simulink model "controllReal"  (R2018a)
settings: Solver=VariableStepAuto  StartTime=0.0  StopTime=1000  RelTol=1e-3
values from neighbouring files (symbols this model uses):
  a = 0.17    [Lab1.m]
  A = 33    [Lab1.m]
  g = 981    [Lab1.m]
  h = 5:1:15    [Lab1.m]
  h0 = 3.2    [Lab1.m]
  hV = [1.826, 2.539, 3.452, 4.18, 4.99, 5.762, 6.665, 7.36, 8.193, 8.93, 9.66]    [Lab1.m]
  v = 1:1:10    [Lab1.m]
  vt = [21.18, 26.66 30.97, 34.28, 37.92, 39.73, 42.53, 45.45, 46.49, 47.67]    [Lab1.m]
undefined symbols (not defined in the file or in its folder): National_Instruments, PCI, sigbuilder_block
libraries: sldrtlib x2
settings Model: Creator=scofre-5  LastModifiedBy=scofre-5

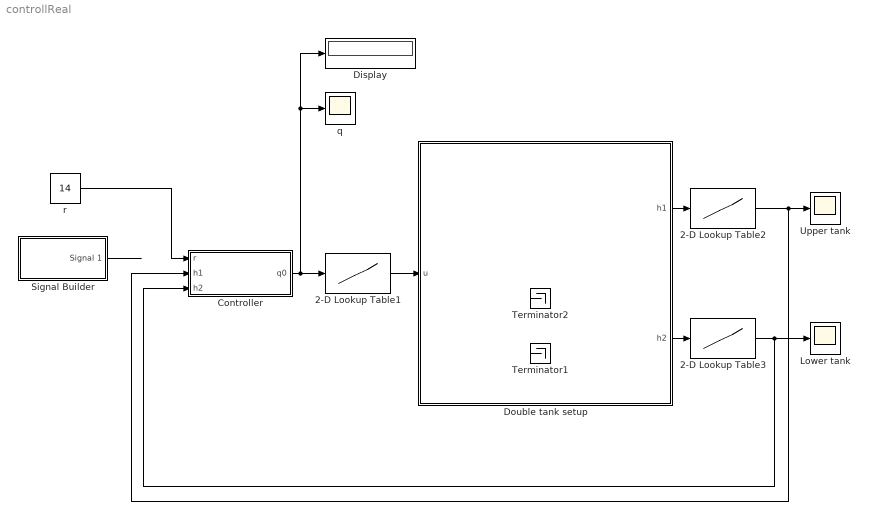
== system controllReal ==
  2-D Lookup Table1 : Lookup_n-D  NumberOfTableDimensions=1  BreakpointsForDimension1=x  BreakpointsForDimension2=[1:3]  Table=y  RndMeth=Simplest  InputSameDT=on  mask{x=v, y=vt}
      mask prompts: x "Values on x-axis"; y "Values on y-axis"
  2-D Lookup Table2 : Lookup_n-D  NumberOfTableDimensions=1  BreakpointsForDimension1=x  BreakpointsForDimension2=[1:3]  Table=y  RndMeth=Simplest  InputSameDT=on  mask{x=hV, y=h}
      mask prompts: x "Values on x-axis"; y "Values on y-axis"
  2-D Lookup Table3 : Lookup_n-D  NumberOfTableDimensions=1  BreakpointsForDimension1=x  BreakpointsForDimension2=[1:3]  Table=y  RndMeth=Simplest  InputSameDT=on  mask{x=hV, y=h}
      mask prompts: x "Values on x-axis"; y "Values on y-axis"
  Controller : Subsystem
  Display : Display
  Double tank setup : Subsystem  AncestorBlock=R0002E_lib/Double tank setup  StopFcn=|  mask(Realtime interface for the tank process){ts=0.02, h1_ch=0, h2_ch=1, u_ch=0}
      | chn =get_param(gcb,'u_ch');                          
      | s = daq.createSession('ni');                         
      | channel = ['ao',chn];                                
      | s.addAnalogOutputChannel('Dev1', channel, 'Voltage');
      | x = zeros(5,1);                                      
      | s.queueOutputData(x);                                
      | lh = s.addlistener('DataRequired', ...               
      | @(src,event) src.queueOutputData(x));                
      | s.startBackground();                                 
      | s.wait();                                            
      | s.stop();                                            
      | delete(lh);                                          
      | clear chn;                                           
      | clear s;                                             
      | clear channel;                                       
      | clear lh;                                            
      | clear x;
      mask prompts: ts "Sample time"; h1_ch "A/D Channel for upper tank"; h2_ch "A/D Channel for lower tank"; u_ch "D/A Channel for pump"
      mask help:
      | This block represents the physical interface from the computer to the tank process.
      |
      | The input u is the voltage that is provided for the pump, the output h1 is the measured level in the upper tank in [V] and the output h2 is the
      | measured level in the lower tank in [V].
      |
      | You need to provide the sample rate at which the voltage to the pump is updated and the level measurements are sampled. The sample rate should not be less than 0.02 seconds.
      mask Display:
      | x=363;
      | y=381;
      | image(imread('tank_icon.jpg'));
      | text(250/x,309/y,'Sensor');
      | text(260/x,169/y,'Sensor');
      | text(335/x,289/y,'A');
      | text(351/x,283/y,'D');
      | text(335/x,100/y,'A');
      | text(351/x,95/y,'D');
      | text(22/x,187/y,'A');
      | text(5/x,195/y,'D');
      | text(225/x,278/y,'h_1','texmode','on');
      | text(225/x,146/y,'h_2','texmode','on');
      | text(300/x,270/y,sprintf('AI-%d',h1_ch));
      | text(300/x,80/y,sprintf('AI-%d',h2_ch));
      | text(40/x,173/y,sprintf('AO-%d',u_ch));
  Lower tank : Scope
  Signal Builder : Subsystem  Tag=STV Subsys  LoadFcn=sigbuilder_block('load');  StartFcn=sigbuilder_block('start');  StopFcn=sigbuilder_block('stop');  ClipboardFcn=sigbuilder_block('clipboard');  mask(Sigbuilder block){tuvar=[0:10]}
      mask help: Simulink:masks:SigbuilderBlock_MD
      mask init:
      | if ~strcmp(get_param(bdroot(gcbh),'SimulationStatus'),'stopped') tuvar = sigbuilder_block('maskInit'); end
      settings: CopyFcn=sigbuilder_block('copy');  DeleteFcn=sigbuilder_block('delete');  ModelCloseFcn=sigbuilder_block('modelClose');  PreSaveFcn=sigbuilder_block('preSave');  PauseFcn=sigbuilder_block('pause');  ContinueFcn=sigbuilder_block('continue');  NameChangeFcn=sigbuilder_block('namechange');  OpenFcn=sigbuilder_block('open',[273 267 483.75 400.5 ]);  CloseFcn=sigbuilder_block('close');
      mask Display: plot(0, 0, 100, 100,[2, 2, 32, 32, 2], [68, 8, 8, 68, 68],[32, 2], [38, 38], [32, 19, 2],[53, 60, 44], [32, 17, 17, 2],[16, 16, 31, 31]);txt = getActiveGroup(gcbh);text(2, 100, txt,'verticalAlignment', 'top');
  Terminator1 : Terminator
  Terminator2 : Terminator
  Upper tank : Scope
  q : Scope
  r : Constant  Value=14
  wires:
  Signal Builder/1(Signal 1) -> ?
  Controller/1(q0) -> 2-D Lookup Table1/1, q/1, Display/1
  2-D Lookup Table1/1 -> Double tank setup/1(u)
  Double tank setup/1(h1) -> 2-D Lookup Table2/1
  Double tank setup/2(h2) -> 2-D Lookup Table3/1
  2-D Lookup Table3/1 -> Controller/3(h2), Lower tank/1
  2-D Lookup Table2/1 -> Controller/2(h1), Upper tank/1
  r/1 -> Controller/1(r)

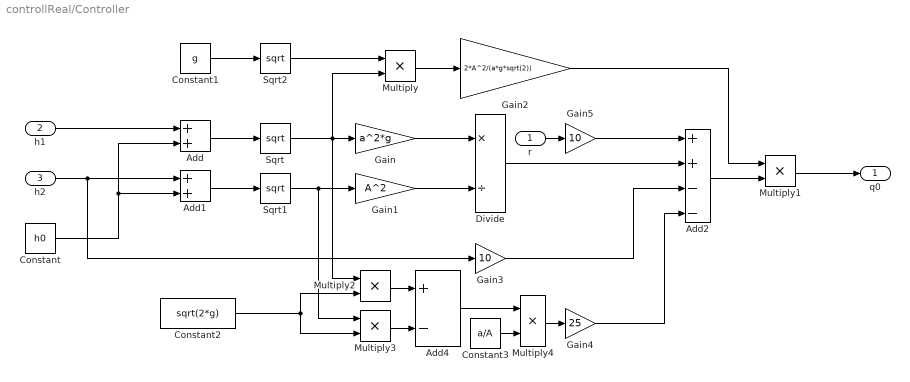
== system controllReal/Controller ==
  r : Inport
  h1 : Inport  Port=2
  h2 : Inport  Port=3
  Add : Sum
  Add1 : Sum
  Add2 : Sum  Inputs=++--
  Add4 : Sum  Inputs=+-
  Constant : Constant  Value=h0
  Constant1 : Constant  Value=g
  Constant2 : Constant  Value=sqrt(2*g)
  Constant3 : Constant  Value=a/A
  Divide : Product  Inputs=*/
  Gain : Gain  Gain=a^2*g
  Gain1 : Gain  Gain=A^2
  Gain2 : Gain  Gain=2*A^2/(a*g*sqrt(2))
  Gain3 : Gain  Gain=10
  Gain4 : Gain  Gain=25
  Gain5 : Gain  Gain=10
  Multiply{,1..4} (5 alike) : Product
  Sqrt : Sqrt  SaturateOnIntegerOverflow=on
  Sqrt1 : Sqrt  SaturateOnIntegerOverflow=on
  Sqrt2 : Sqrt  SaturateOnIntegerOverflow=on
  q0 : Outport
  wires:
  Constant/1 -> Add1/2, Add/2
  h1/1 -> Add/1
  h2/1 -> Gain3/1, Add1/1
  Add/1 -> Sqrt/1
  Add1/1 -> Sqrt1/1
  Constant1/1 -> Sqrt2/1
  Sqrt/1 -> Multiply/2, Multiply2/1, Gain/1
  Sqrt1/1 -> Multiply3/1, Gain1/1
  Gain/1 -> Divide/1
  Gain1/1 -> Divide/2
  Divide/1 -> Add2/2
  r/1 -> Gain5/1
  Sqrt2/1 -> Multiply/1
  Multiply/1 -> Gain2/1
  Add2/1 -> Multiply1/2
  Gain2/1 -> Multiply1/1
  Multiply1/1 -> q0/1
  Gain3/1 -> Add2/3
  Constant2/1 -> Multiply3/2, Multiply2/2
  Multiply2/1 -> Add4/1
  Multiply3/1 -> Add4/2
  Add4/1 -> Multiply4/1
  Constant3/1 -> Multiply4/2
  Multiply4/1 -> Gain4/1
  Gain4/1 -> Add2/4
  Gain5/1 -> Add2/1

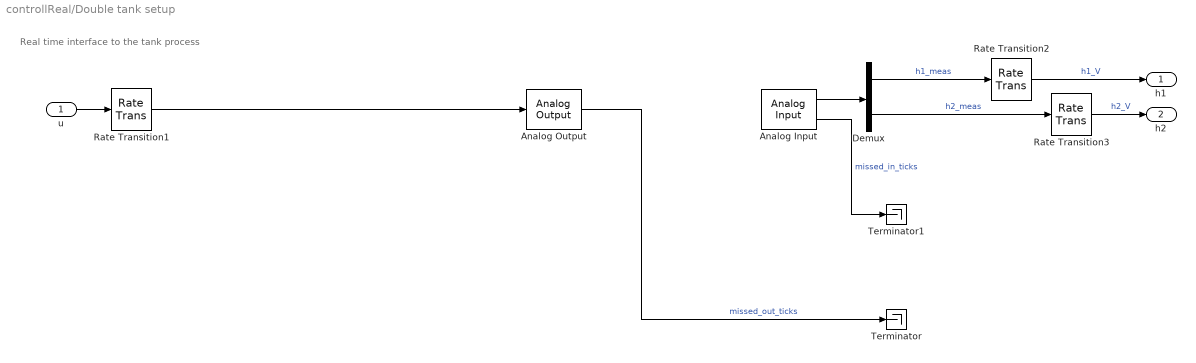
== system controllReal/Double tank setup ==
  note: Real time interface to the tank process
  u : Inport
  Analog Input : sldrtlib/Analog Input  SampleTime=ts  MaxMissedTicks=500000000  ShowMissedTicks=on  YieldWhenWaiting=off  DrvName=National_Instruments/PCI-6024E  DrvAddress=4294967295  DrvOptions=[0 0 0 0 0 0]  Channels=[h1_ch+1,h2_ch+1]  RangeMode=1  VoltRange=1  DataType=1
      settings: AttributesFormatString=National Instruments\nPCI-6024E [auto]  SourceProductName=Simulink Desktop Real-Time
  Analog Output : sldrtlib/Analog Output  SampleTime=ts  MaxMissedTicks=500000000  ShowMissedTicks=on  YieldWhenWaiting=off  DrvName=National_Instruments/PCI-6024E  DrvAddress=4294967295  DrvOptions=[0 0 0 0 0 0]  Channels=u_ch+1  RangeMode=1  VoltRange=1  InitialValue=0  FinalValue=0
      settings: AttributesFormatString=National Instruments\nPCI-6024E [auto]  SourceProductName=Simulink Desktop Real-Time
  Demux : Demux  Outputs=2
  Rate Transition1 : RateTransition  OutPortSampleTime=ts
  Rate Transition2 : RateTransition
  Rate Transition3 : RateTransition
  Terminator : Terminator
  Terminator1 : Terminator
  h1 : Outport
  h2 : Outport  Port=2
  wires:
  Rate Transition1/1 -> Analog Output/1
  Rate Transition3/1 -> h2/1  "h2_V"
  Rate Transition2/1 -> h1/1  "h1_V"
  Analog Input/2 -> Terminator1/1  "missed_in_ticks"
  Demux/2 -> Rate Transition3/1  "h2_meas"
  Demux/1 -> Rate Transition2/1  "h1_meas"
  Analog Input/1 -> Demux/1
  Analog Output/1 -> Terminator/1  "missed_out_ticks"
  u/1 -> Rate Transition1/1

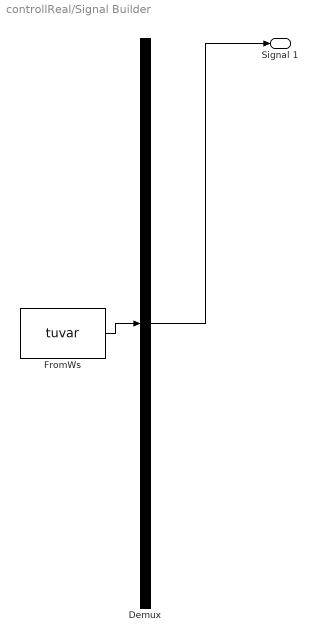
== system controllReal/Signal Builder ==
  Demux : Demux  Tag=STV Demux  Outputs=1
  FromWs : FromWorkspace  Tag=STV FromWs  VariableName=tuvar  SampleTime=0
      SigBuilderData=|
      | common.afterFinalStr = 'Extrapolate'
      | common.sampleTime = 0
      | dataSet.timeRange = [0 60]
      | dataSet.name = 'Group 1'
      | sbobj.Groups.Name = 'Group 1'
      | sbobj.Groups.Signals.Name = 'Signal 1'
      | sbobj.Groups.Signals.XData = [0 4 20 40 58 60]
      | sbobj.Groups.Signals.YData = [0 0 7 1 5 5]
      | sbobj.Groups.TimeRange = [0 60]
  Signal 1 : Outport  Tag=STV Outport
  wires:
  Demux/1 -> Signal 1/1
  FromWs/1 -> Demux/1
